simulink library "carnot"  (R2018b)
settings: Solver=VariableStepAuto  StartTime=0.0  StopTime=10.0  RelTol=1e-3
undefined symbols (not defined in the file or in its folder): A, A_earth, acol, Acol, ActPower1, ActPower2, ActPower3, Ad, Ad0, Ar, Au, Au0, Azimuth_Angle, B, Bd, Bd0, Br, Bu, Bu0, C, c1, c2, c3, c33, c4, c5, c6, CarnotCallbacks_Density, CarnotCallbacks_Enthalpy, CarnotCallbacks_Enthalpy2Temperature, CarnotCallbacks_Entropy, CarnotCallbacks_Evaporation_Enthalpy, CarnotCallbacks_GlobalMessageLevel, CarnotCallbacks_Grashof, CarnotCallbacks_Heat_Capacity, CarnotCallbacks_Kinematic_Viscosity, CarnotCallbacks_PMV_PPD, CarnotCallbacks_Prandtl, CarnotCallbacks_Saturation_Property, CarnotCallbacks_Saturation_Temperature, CarnotCallbacks_Saturation_Value_Water, CarnotCallbacks_Specific_Volume, CarnotCallbacks_Thermal_Conductivity, CarnotCallbacks_Vapour_Content, CarnotCallbacks_Vapour_Pressure, Cd, Cdl, Cr, Cu, Davies, Dd, DE_TRY2010_04_averageYear, delta_grd, density, DiameterLastPiece, dl, DPConstant, DPLinear, DPQuadratic, Dr ... (+59)
libraries: $bdroot x429, simulink x36, simulink_extras x12
(part 22 of 22)

== system carnot/Source/Chiller/Cooling_Tower/Leistungseinflüsse // influence on coolingpower/t_ia_ist  ==
  Qdot_i_ist : Inport
  t_ie : Inport  Port=2
  cp_i : Inport  Port=3
  mdot : Inport  Port=4
  Add : Sum  Inputs=-+
  Divide : Product  Inputs=*//
  Divide1 : Product  Inputs=*/
  isinf : MATLAB Function  TreatAsAtomicUnit=on
  isnan : MATLAB Function  TreatAsAtomicUnit=on
  phi_Le2 : Constant  Value=1000
  t_ia_ist : Outport
  wires:
  Add/1 -> t_ia_ist/1
  Qdot_i_ist/1 -> Divide/1
  t_ie/1 -> Add/2
  Divide/1 -> isnan/1(u)
  cp_i/1 -> Divide1/1
  isnan/1(y) -> isinf/1(u)
  phi_Le2/1 -> Divide1/2
  Divide1/1 -> Divide/2
  mdot/1 -> Divide/3
  isinf/1(y) -> Add/1

== system carnot/Source/Chiller/Cooling_Tower/Verbrauch // consumption/Strom ==
  control_Fan : Inport
  P_Fan : Inport  Port=2
  Add : Sum
  Integrator1 : Integrator
  Product : Product  RndMeth=Zero
  Product2 : Product  Inputs=*/  SaturateOnIntegerOverflow=on  RndMeth=Zero  InputSameDT=on  OutDataTypeStr=Inherit: Same as first input
  Rieselwasserpumpe [kW] : Constant  Value=0.25
  factor1 : Constant  Value=3600
  energy : Outport
  power : Outport  Port=2
  wires:
  Rieselwasserpumpe [kW]/1 -> Add/1
  Product/1 -> power/1, Integrator1/1
  control_Fan/1 -> Product/1
  Add/1 -> Product/2
  P_Fan/1 -> Add/2
  Integrator1/1 -> Product2/1
  factor1/1 -> Product2/2
  Product2/1 -> energy/1

== system carnot/Source/Chiller/Cooling_Tower/Verbrauch // consumption/Verdunstung ==
  control_Fan : Inport
  t_le : Inport  Port=2
  phi_le : Inport  Port=3
  Vdot_Fan : Inport  Port=4
  Qdot : Inport  Port=5
  t_ie : Inport  Port=6
  "Enthalpie " : Subsystem
  Integrator1 : Integrator
  Product : Product  RndMeth=Zero
  Product1 : Product  RndMeth=Zero
  Product2 : Product  Inputs=*/  SaturateOnIntegerOverflow=on  RndMeth=Zero  InputSameDT=on  OutDataTypeStr=Inherit: Same as first input
  Product3 : Product  RndMeth=Zero
  RelHum2x : $bdroot/Basic/Material_Properties/RelHum2x
  Saturation_Temperature : $bdroot/Basic/Material_Properties/Saturation_Temperature  VariantControl=CarlibClassic  INPUTARGUMENTS=state variables (classic)  DEBUGLEVEL=WARNINGLEVEL  MAXTOTALMESSAGES=inf  MAXCONSECUTIVEMESSAGES=inf  WRITETOFILE=0  FILENAME='errors.txt'
  Verdunstungsmenge : MATLAB Function  TreatAsAtomicUnit=on
  air : Constant  Value=2
  factor1 : Constant  Value=3600
  p : Constant  Value=1e5
  roh_air : Constant  Value=1.29
  Wasserverbrauch : Outport
  wires:
  t_le/1 -> RelHum2x/1, Saturation_Temperature/1, "Enthalpie "/2(t_le)
  p/1 -> RelHum2x/2, Saturation_Temperature/2, Verdunstungsmenge/7(p)
  phi_le/1 -> RelHum2x/3
  Vdot_Fan/1 -> Product/1
  roh_air/1 -> Product/2
  "Enthalpie "/1(h_le) -> Verdunstungsmenge/1(h_le)
  RelHum2x/1 -> "Enthalpie "/1(x_le), Saturation_Temperature/4, Verdunstungsmenge/5(x_le)
  Qdot/1 -> Verdunstungsmenge/3(qdot)
  Saturation_Temperature/1 -> Verdunstungsmenge/6(t_tau)
  air/1 -> Saturation_Temperature/3
  Integrator1/1 -> Product2/1
  factor1/1 -> Product2/2
  Product2/1 -> Wasserverbrauch/1
  Product1/1 -> Integrator1/1
  control_Fan/1 -> Product1/1
  Product3/1 -> Product1/2
  Product/1 -> Verdunstungsmenge/2(mdot), Product3/1
  t_ie/1 -> Verdunstungsmenge/4(t_ie)
  Verdunstungsmenge/1(x_fl) -> Product3/2

== system carnot/Source/Cogeneration/microCHP_constant/pump and return temperature raising facility/heat capacity ==
  Tin : Inport
  heat capacity : StateSpace  A=-NTU  B=NTU  D=0  InitialCondition=80
  T : Outport
  wires:
  Tin/1 -> heat capacity/1
  heat capacity/1 -> T/1

== system carnot/Source/Cogeneration/microCHP_modulating/pump_const/heat capacity ==
  Tin : Inport
  heat capacity : StateSpace  A=-NTU  B=NTU  D=0  InitialCondition=80
  T : Outport
  wires:
  heat capacity/1 -> T/1
  Tin/1 -> heat capacity/1

== system carnot/Source/Heat_Pump/Ground_Source_Heat_Exchanger/BoundaryCondition2/g-function ==
  note: temperature funnel: 1/(2*pi*lambdaErde)
  note: operation time, limited to 1 s (avoid division by zero)
  qdot,i : Inport
  Bias : Bias  Bias=t_start
  Clock : Clock
  Constant1 : Constant
  Constant2 : Constant
  Dd2 : Gain  Gain=1/(2*pi*lambdaErde)  SaturateOnIntegerOverflow=on  OutDataTypeStr=Inherit: Same as input  ParamDataTypeStr=Inherit: Same as input
  Integrator : Integrator
  Integrator1 : Integrator  LowerSaturationLimit=1
  Max : MinMax  Function=max  Inputs=2
  Product : Product  Inputs=/**  SaturateOnIntegerOverflow=on  RndMeth=Zero  InputSameDT=on  OutDataTypeStr=Inherit: Same as first input
  RechenRadius : Constant  Value=Rechenradius  VectorParams1D=off
  Squeeze : Squeeze
  deltaT : Scope  Commented=on
  g-function : Lookup_n-D  BreakpointsForDimension1=t_Trichter  BreakpointsForDimension2=r_Trichter  BeginIndexSearchUsingPreviousIndexResult=on  Table=gfunction  InternalRulePriority=Speed  RndMeth=Simplest  InputSameDT=on
  g-values : Scope  Commented=on
  DeltaT : Outport
  wires:
  Bias/1 -> g-function/1
  Clock/1 -> Bias/1
  Constant2/1 -> Integrator1/1
  Max/1 -> Product/1  "operation time"
  Constant1/1 -> Max/2
  Integrator1/1 -> Max/1
  Integrator/1 -> Product/2  "energy per meter"
  Squeeze/1 -> Dd2/1
  qdot,i/1 -> Integrator/1  "power per meter"
  g-function/1 -> Squeeze/1, g-values/1
  Product/1 -> DeltaT/1, deltaT/1
  Dd2/1 -> Product/3
  RechenRadius/1 -> g-function/2

== system carnot/Source/Solar_Thermal/Collector_Unglazed/Collector_Unglazed/create_Cdat ==
  acol : Inport
  THBin : Inport  Port=2
  THBout : Inport  Port=3
  Qdot : Inport  Port=4
  Tmean : Inport  Port=5
  WDB : Inport  Port=6
  Bus Creator : BusCreator  Inputs=6
  data_c : Outport
  wires:
  acol/1 -> Bus Creator/1  "Acol"
  THBin/1 -> Bus Creator/2  "THBin"
  THBout/1 -> Bus Creator/3  "THBout"
  WDB/1 -> Bus Creator/6  "WDB_surface"
  Bus Creator/1 -> data_c/1
  Qdot/1 -> Bus Creator/4  "Qdot"
  Tmean/1 -> Bus Creator/5  "Tmean"

== system carnot/Source/Solar_Thermal/SolarCollector_2node/glazed_collector_ISO9806/Tin_node ==
  note: CapAbs/2 * dT/dt = mdot*cp*(Tin-T)
  A : Inport
  THB : Inport  Port=2
  Bus Assignment : BusAssignment  AssignedSignals=Temperature
  Bus Selector5 : BusSelector  OutputSignals=Temperature,MassFlow
  Gain : Gain  Gain=2
  Integrator : Integrator  InitialCondition=tini
  Product2 : Product  Inputs=3  RndMeth=Zero
  Product4 : Product  Inputs=*//  RndMeth=Zero
  Subtract3 : Sum  Inputs=-+
  c_abs : Constant  Value=c5
  heat_capacity : $bdroot/Basic/Material_Properties/Heat_Capacity  VariantControl=CarlibClassic  INPUTARGUMENTS=THB  DEBUGLEVEL=DEBUGLEVEL  MAXTOTALWARNINGS=inf  MAXCONSECUTIVEWARNINGS=inf  WRITETOFILE=0  FILENAME='errors.txt'
  THB_ : Outport
  wires:
  Product4/1 -> Integrator/1
  THB/1 -> heat_capacity/1, Bus Selector5/1, Bus Assignment/1
  Bus Assignment/1 -> THB_/1
  heat_capacity/1 -> Product2/3
  Bus Selector5/1 -> Subtract3/2  "<Temperature>"
  Bus Selector5/2 -> Product2/2  "<MassFlow>"
  Subtract3/1 -> Product2/1
  Product2/1 -> Gain/1  "power"
  Gain/1 -> Product4/1
  Integrator/1 -> Bus Assignment/2, Subtract3/1  "Tsol"
  c_abs/1 -> Product4/2
  A/1 -> Product4/3

== system carnot/Storage/Thermal/Storage_Ports/Pipe_stratified/T_criteria not satisfied ==
  Action Port : ActionPort
  MATLAB Fcn1 : MATLABFcn  MATLABFcn=[zeros(u-1,1); 1; zeros(nodes-u,1)]  OutputDimensions=nodes
  const : Constant  Value=outlet
  Out1 : Outport  OutputWhenDisabled=reset  InitialOutput=0
  wires:
  const/1 -> MATLAB Fcn1/1
  MATLAB Fcn1/1 -> Out1/1

== system carnot/Storage/Thermal/Storage_Ports/Pipe_stratified/massflow downwards ==
  In1 : Inport
  Action Port : ActionPort
  MATLAB Fcn : MATLABFcn  MATLABFcn=find(u,1,'last')+outlet-1  OutputDimensions=1
  MATLAB Fcn1 : MATLABFcn  MATLABFcn=[zeros(u-1,1); 1; zeros(nodes-u,1)]  OutputDimensions=nodes
  Out1 : Outport
  wires:
  MATLAB Fcn/1 -> MATLAB Fcn1/1
  In1/1 -> MATLAB Fcn/1
  MATLAB Fcn1/1 -> Out1/1

== system carnot/Storage/Thermal/Storage_Ports/Pipe_stratified/massflow upwards ==
  In1 : Inport
  Action Port : ActionPort
  MATLAB Fcn : MATLABFcn  MATLABFcn=find(u,1,'first')+inlet-1  OutputDimensions=1
  MATLAB Fcn1 : MATLABFcn  MATLABFcn=[zeros(u-1,1); 1; zeros(nodes-u,1)]  OutputDimensions=nodes
  Out1 : Outport
  wires:
  In1/1 -> MATLAB Fcn/1
  MATLAB Fcn/1 -> MATLAB Fcn1/1
  MATLAB Fcn1/1 -> Out1/1

== system carnot/Storage/Thermal/surface_models/Open_Surface/add 5.6 ==
  In1 : Inport
  Sum : Sum  SaturateOnIntegerOverflow=on  InputSameDT=on  OutDataTypeStr=Inherit: Same as first input
  const : Constant  Value=c
  Out1 : Outport
  wires:
  const/1 -> Sum/1
  In1/1 -> Sum/2
  Sum/1 -> Out1/1

== system carnot/Basic/Thermal_Models/Room_Node/convective_node/PressureCalculation/Subsystem ==
  note: (J/(kg*K)
  T : Inport
  Celsius2Kelvin : Bias  Bias=273.15
  air_gas_constant : Gain  Gain=287  SaturateOnIntegerOverflow=on  OutDataTypeStr=Inherit: Same as input  ParamDataTypeStr=Inherit: Same as input
  R*T ' : Outport
  wires:
  Celsius2Kelvin/1 -> air_gas_constant/1
  T/1 -> Celsius2Kelvin/1
  air_gas_constant/1 -> R*T '/1

== system carnot/Source/Chiller/Cooling_Tower/Verbrauch // consumption/Verdunstung/Enthalpie  ==
  x_le : Inport
  t_le : Inport  Port=2
  Add : Sum
  Add1 : Sum
  Product : Product  RndMeth=Zero
  Product1 : Product  RndMeth=Zero
  Product2 : Product  RndMeth=Zero
  cp_d : Constant  Value=1.861
  cp_lt : Constant  Value=1.006
  dhv0 : Constant  Value=2500
  h_le : Outport
  wires:
  Add/1 -> h_le/1
  cp_lt/1 -> Product/1
  t_le/1 -> Product/2, Product2/1
  Product/1 -> Add/1
  Product1/1 -> Add/2
  x_le/1 -> Product1/1
  cp_d/1 -> Product2/2
  Add1/1 -> Product1/2
  Product2/1 -> Add1/1
  dhv0/1 -> Add1/2

== matlab function carnot/Source/Chiller/Absorption_Chiller_LookUp/cooling/isinf ==
  data: u input; y output

function y = fcn(u)

%Verhindert die Fehlerausgabe bei Teilen mit dem Wert 0 
%Dieser Zustand tritt ein wenn der Volumenstrom 0 l/s gesetzt wird.

v = isinf (u);

if v == 0
    
    y = u;

else 
    
    y = 0;
    
end

== matlab function carnot/Source/Chiller/Absorption_Chiller_LookUp/cooling/isnan ==
  data: u input; y output

function y = fcn(u)

%Verhindert die Fehlerausgabe bei Teilen durch den Wert 0 
%Dieser Zustand tritt ein wenn der Volumenstrom 0 l/s gesetzt wird.

v = isnan (u);

if v == 0
    
    y = u;

else 
    
    y = 0;
    
end

== matlab function carnot/Source/Chiller/Absorption_Chiller_LookUp/generator/isinf ==
  data: u input; y output

function y = fcn(u)

%Verhindert die Fehlerausgabe bei Teilen mit dem Wert 0 
%Dieser Zustand tritt ein wenn der Volumenstrom 0 l/s gesetzt wird.

v = isinf (u);

if v == 0
    
    y = u;

else 
    
    y = 0;
    
end

== matlab function carnot/Source/Chiller/Cooling_Tower/Feuchtkugel- temperatureinfluss // wet-bulb temperature effect/Abgleich /Embedded MATLAB Function ==
  data: t_fk input; y output; t_ia_fk15 input; t_ie input
%Festlegung der Eingänge
function y = fcn(t_fk, t_ia_fk15, t_ie)

%Änderung des Faktors
if t_ie < 41
    
    y = ((t_fk-15)*0.27)+t_ia_fk15;
    
else
    
    y = ((t_fk-15)*0.25)+t_ia_fk15;
    
end

== matlab function carnot/Source/Chiller/Absorption_Chiller_LookUp/generator/isnan ==
  data: u input; y output

function y = fcn(u)

%Verhindert die Fehlerausgabe bei Teilen durch den Wert 0 
%Dieser Zustand tritt ein wenn der Volumenstrom 0 l/s gesetzt wird.

v = isnan (u);

if v == 0
    
    y = u;

else 
    
    y = 0;
    
end

== matlab function carnot/Source/Chiller/Absorption_Chiller_LookUp/recooling/isinf ==
  data: u input; y output

function y = fcn(u)

%Verhindert die Fehlerausgabe bei Teilen mit dem Wert 0 
%Dieser Zustand tritt ein wenn der Volumenstrom 0 l/s gesetzt wird.

v = isinf (u);

if v == 0
    
    y = u;

else 
    
    y = 0;
    
end

== matlab function carnot/Source/Chiller/Absorption_Chiller_LookUp/recooling/isnan ==
  data: u input; y output

function y = fcn(u)

%Verhindert die Fehlerausgabe bei Teilen durch den Wert 0 
%Dieser Zustand tritt ein wenn der Volumenstrom 0 l/s gesetzt wird.

v = isnan (u);

if v == 0
    
    y = u;

else 
    
    y = 0;
    
end

== matlab function carnot/Source/Chiller/Cooling_Tower/Leistungseinflüsse // influence on coolingpower/t_ia_ist /isinf ==
  data: u input; y output

function y = fcn(u)

%Verhindert die Fehlerausgabe bei Teilen mit dem Wert 0 
%Dieser Zustand tritt ein wenn der Volumenstrom 0 l/s gesetzt wird.

v = isinf (u);

if v == 0
    
    y = u;

else 
    
    y = 0;
    
end

== matlab function carnot/Source/Chiller/Cooling_Tower/Leistungseinflüsse // influence on coolingpower/t_ia_ist /isnan ==
  data: u input; y output

function y = fcn(u)

%Verhindert die Fehlerausgabe bei Teilen durch den Wert 0 
%Dieser Zustand tritt ein wenn der Volumenstrom 0 l/s gesetzt wird.

v = isnan (u);

if v == 0
    
    y = u;

else 
    
    y = 0;
    
end

== matlab function carnot/Source/Chiller/Cooling_Tower/Verbrauch // consumption/Verdunstung/Verdunstungsmenge ==
  data: h_le input; mdot input; x_fl output; qdot input; t_ie input; x_le input; t_tau input; p input
function x_fl = fcn(h_le, mdot, qdot, t_ie, x_le, t_tau, p)

cp_lt = 1.006;
cp_d = 1.861;
cp_w = 4.19;
dhv0 = 2500;
tmax = t_ie;
tmin = t_tau;
t_zw = 15;
phi_luftaus = 100;
m = 1;


% Vorbedingung qdot muss positiv sein um eine Verdunstung zu gewährleisten ansonsten ist es ein Kondensation
if qdot < 0
    
    x_luftaus = 0;
    
else
    % Luftaustrittstemperaturberechnung, Halbierungsverfahren
        t_luftaus = (tmax+tmin)/2;
    
    % Absolute Feuchte-Berechnung Lufteintritt
        ps_luftaus = 611*exp((-1.91275)*10^(-4)+7.258*10^(-2)*t_luftaus-2.939*10^(-4)*t_luftaus^2+9.841*10^(-7)*t_luftaus^3-1.92*10^(-9)*t_luftaus^4);
        x_luftaus = (0.622*(phi_luftaus/100)*ps_luftaus)/(p-(phi_luftaus/100)*ps_luftaus);

    % Enthalpie Luftaustritt mit dem schon berechneten Qpkt
        h_la = qdot/mdot + (x_luftaus-x_le)*cp_w*t_zw + h_le;
    
    % Austrittstemperatur 
        tlab = (h_la - x_luftaus*dhv0)/(cp_lt + x_luftaus*cp_d);

    % Beginn der Schleife 
    % (t_luftaus - tlab) < 0,001 und > -0,001 ist die Austrittstemperatur gefunden
    %  t_luftaus < tlab  tmin = t_luftaus
    %  t_luftaus > tlab  tmax = t_luftaus
        while (t_luftaus - tlab)>0.001 || (t_luftaus - tlab) < -0.001 && m < 30
    
            if t_luftaus < tlab
        
                tmin = t_luftaus;
    
            else
        
                tmax = t_luftaus;
    
            end
    
            % Luftaustrittstemperaturberechnung, Halbierungsverfahren
                t_luftaus = (tmax+tmin)/2;
    
            % Absolute Feuchte-Berechnung Lufteintritt
                ps_luftaus = 611*exp((-1.91275)*10^(-4)+7.258*10^(-2)*t_luftaus-2.939*10^(-4)*t_luftaus^2+9.841*10^(-7)*t_luftaus^3-1.92*10^(-9)*t_luftaus^4);
                x_luftaus = (0.622*(phi_luftaus/100)*ps_luftaus)/(p-(phi_luftaus/100)*ps_luftaus);
        
            % Enthalpie Luftaustritt mit dem schon berechneten Qpkt
                h_la = qdot/mdot + (x_luftaus-x_le)*cp_w*t_zw + h_le;
        
            % Austrittstemperatur 
                tlab = (h_la - x_luftaus*dhv0)/(cp_lt + x_luftaus*cp_d);
        
            % Schleifenzähler
                m = m + 1;
    
        end

end

x_fl = x_luftaus-x_le;

== matlab function carnot/Source/Chiller/Compression_Air_Water_Chiller/cooling/isinf ==
  data: u input; y output

function y = fcn(u)

% Avoids errors when dividing by very small values. 
% This situation appears when the massflow is near zero.

v = isinf (u);

if v == 0
    
    y = u;

else 
    
    y = 0;
    
end

== matlab function carnot/Source/Chiller/Compression_Air_Water_Chiller/cooling/isnan ==
  data: u input; y output

function y = fcn(u)

% Avoids errors when dividing by zero. 
% This situation appears when the massflow is zero.

v = isnan (u);

if v == 0
    
    y = u;

else 
    
    y = 0;
    
end
